simulink model "vehicle_modes"  (R2025b)
settings: Solver=VariableStepAuto  StartTime=0.0  StopTime=100  RelTol=1e-3
model workspace (MAT data in the model file):
  Bmax = 6000
  Cd = 0.32
  Cr = 0.015
  M = 1200
  Tmax = 250
  mode_cm = 2
  mode_cmd = 3
  mode_command = 3
  p_row = 1.225
  radius = 0.3
settings Model: Creator=10870  LastModifiedBy=10870

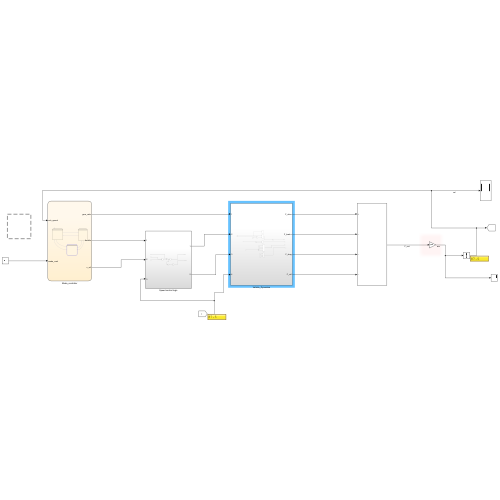
[thumbnail: Simulink's stored preview of the top-level diagram]
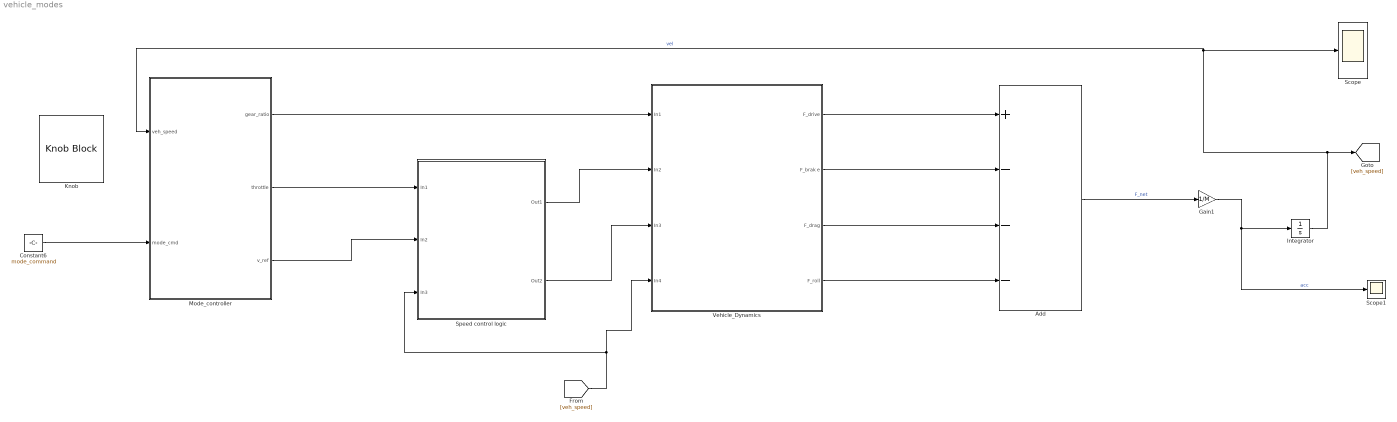
== system vehicle_modes ==
  Add : Sum  Inputs=+---
  Constant6 : Constant  Value=mode_command
  Gain1 : Gain  Gain=1/M
  Integrator : Integrator
  Knob : KnobBlock  ScaleMin=1  ScaleMax=3  TickInterval=1.0000
  Mode_controller : Stateflow chart  TreatAsAtomicUnit=on
      settings: PortSchema="{\"entries\":[{\"content\":{\"sides\":[{\"content\":{\"connectorIds\":[\"In1\",\"In2\"]},\"type\":\"ConnectorPlacement.EquallySpacedRectSide\",\"uuid\":\"0ac8a5aa-c43e-446f-a67b-bdd58b828e81\"},{\"content\":{\"connectorIds\":[\"Out1\",\"Out3\",\"Out2\"],\"side\":\"RIGHT\"},\"type\":\"ConnectorPlacement.EquallySpacedRectSide\",\"uuid\":\"f08d2692-71dd-4472-a357-68dab1029f9a\"},{\"content\":{\"side\":\"TOP\"},\"type\":\"ConnectorPlacement.EquallySpacedRectSide\",\"uuid\":\"037eac55-8252-4c07-a2b4-a64ffa4142e0\"}]},\"type\":\"ConnectorPlacement.EquallySpacedConnector\",\"uuid\":\"3547915d-01a5-474b-8346-df4124959806\"}],\"packageUris\":[\"http://schema.mathworks.com/mf0/Connector/R2020b\"],\"version\":\"1.0\"}"
  Scope : Scope
      settings: ActiveDisplayYMinimum=-89.25314706069193  ActiveDisplayYMaximum=285.04012820290524
  Scope1 : Scope
      settings: ActiveDisplayYMinimum=-7.9408984677471173  ActiveDisplayYMaximum=4.7649753442050633
  Speed control logic : Subsystem
  Vehicle_Dynamics : Subsystem
  wires:
  Gain1/1 -> Scope1/1, Integrator/1  "acc"
  Integrator/1 -> Mode_controller/1(veh_speed), Scope/1, [veh_speed]  "vel"
  [veh_speed] -> Vehicle_Dynamics/4(In4), Speed control logic/3(In3)
  Add/1 -> Gain1/1  "F_net"
  Constant6/1 -> Mode_controller/2(mode_cmd)
  Mode_controller/3(throttle) -> Speed control logic/1(In1)
  Mode_controller/2(v_ref) -> Speed control logic/2(In2)
  Mode_controller/1(gear_ratio) -> Vehicle_Dynamics/1(In1)
  Speed control logic/1(Out1) -> Vehicle_Dynamics/2(In2)
  Speed control logic/2(Out2) -> Vehicle_Dynamics/3(In3)
  Vehicle_Dynamics/1(F_drive) -> Add/1
  Vehicle_Dynamics/2(F_brak e) -> Add/2
  Vehicle_Dynamics/3(F_drag) -> Add/3
  Vehicle_Dynamics/4(F_roll) -> Add/4

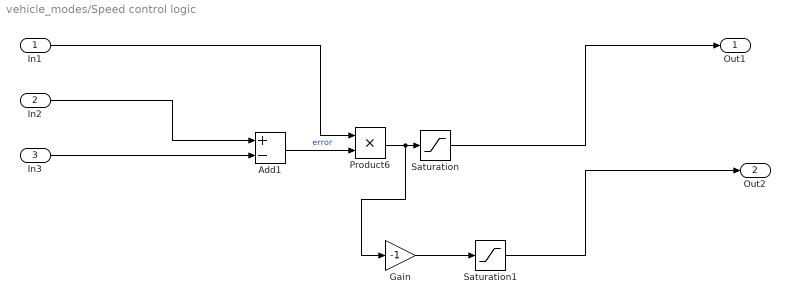
== system vehicle_modes/Speed control logic ==
  In1 : Inport
  In2 : Inport  Port=2
  In3 : Inport  Port=3
  Add1 : Sum  Inputs=+-
  Gain : Gain  Gain=-1
  Product6 : Product
  Saturation : Saturate  UpperLimit=1  LowerLimit=0
  Saturation1 : Saturate  UpperLimit=1  LowerLimit=0
  Out1 : Outport
  Out2 : Outport  Port=2
  wires:
  Add1/1 -> Product6/2  "error"
  Saturation/1 -> Out1/1
  In3/1 -> Add1/2
  Product6/1 -> Gain/1, Saturation/1
  Gain/1 -> Saturation1/1
  In1/1 -> Product6/1
  Saturation1/1 -> Out2/1
  In2/1 -> Add1/1

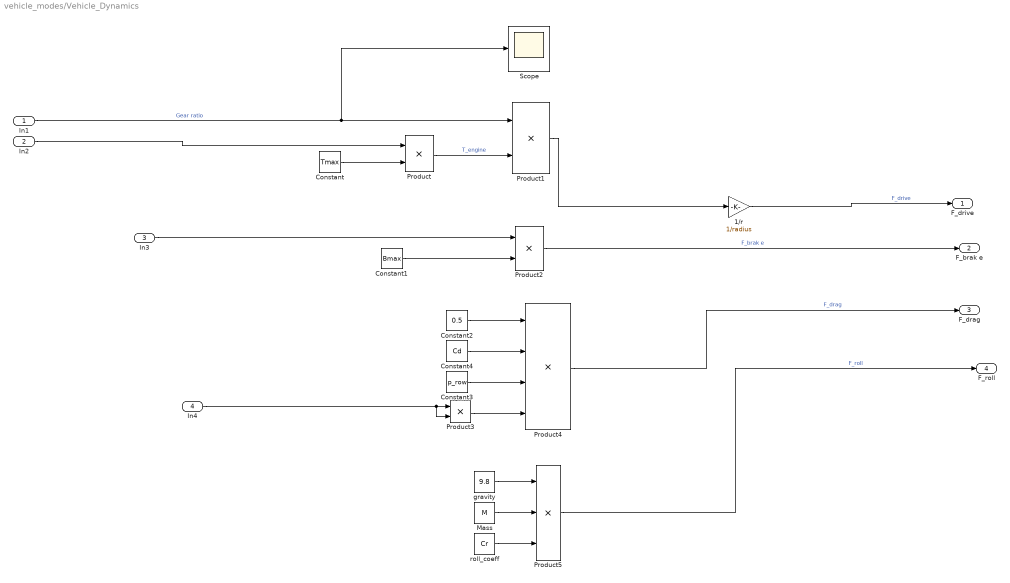
== system vehicle_modes/Vehicle_Dynamics ==
  In1 : Inport
  In2 : Inport  Port=2
  In3 : Inport  Port=3
  In4 : Inport  Port=4
  1/r : Gain  Gain=1/radius
  Constant : Constant  Value=Tmax
  Constant1 : Constant  Value=Bmax
  Constant2 : Constant  Value=0.5
  Constant3 : Constant  Value=p_row
  Constant4 : Constant  Value=Cd
  Mass : Constant  Value=M
  Product{,1..3} (4 alike) : Product
  Product4 : Product  Inputs=4
  Product5 : Product  Inputs=3
  Scope : Scope
      settings: ActiveDisplayYMinimum=-3.3755900316606384  ActiveDisplayYMaximum=8.65750613679479  DataLoggingVariableName=ScopeData2
  gravity : Constant  Value=9.8
  roll_coeff : Constant  Value=Cr
  F_drive : Outport
  F_brak e : Outport  Port=2
  F_drag : Outport  Port=3
  F_roll : Outport  Port=4
  wires:
  Product1/1 -> 1/r/1
  In4/1 -> Product3/2, Product3/1
  Constant4/1 -> Product4/2
  In3/1 -> Product2/1
  Constant3/1 -> Product4/3
  Constant1/1 -> Product2/2
  Mass/1 -> Product5/2
  Constant2/1 -> Product4/1
  In1/1 -> Scope/1, Product1/1  "Gear ratio"
  Constant/1 -> Product/2
  roll_coeff/1 -> Product5/3
  gravity/1 -> Product5/1
  Product3/1 -> Product4/4
  Product2/1 -> F_brak e/1  "F_brak e"
  Product/1 -> Product1/2  "T_engine"
  1/r/1 -> F_drive/1  "F_drive"
  Product5/1 -> F_roll/1  "F_roll"
  Product4/1 -> F_drag/1  "F_drag"
  In2/1 -> Product/1

== stateflow chart vehicle_modes/Mode_controller ==
  state Eco_mode
    en: v_ref = 60
    throttle = 0.4
    during:
    if  veh_speed < 40
    gear_ratio = 4.2;
    elseif veh_speed > 60
    gear_ratio = 2.6;
    else
    gear_ratio = 1.6;
    end
  state Normal_mode
    en: v_ref = 90
    throttle = 0.7
    during: if veh_speed < 40
    gear_ratio = 4.2;
    elseif veh_speed >90
    gear_ratio = 2.6;
    else
    gear_ratio = 1.6;
    end
  state Sport_mode
    en: v_ref = 120;
    throttle = 1.0;
    during: if veh_speed < 50
    gear_ratio = 5.0;
    elseif veh_speed < 100
    gear_ratio = 3.2;
    else
    gear_ratio = 2.0;
    end
  (default) -> Eco_mode
  Eco_mode -> Normal_mode [order 1] : [mode_cmd==2]
  Normal_mode -> Eco_mode [order 1] : [mode_cmd==1]
  Sport_mode -> Eco_mode [order 1] : [mode_cmd==1]
  Eco_mode -> Sport_mode [order 2] : [mode_cmd==3]
  Normal_mode -> Sport_mode [order 2] : [mode_cmd==3]
  Sport_mode -> Normal_mode [order 2] : [mode_cmd==2]
  data: veh_speed input; gear_ratio output; v_ref output; mode_cmd input; throttle output
